simulink model "UScityblock2_Intersection"  (R2021b)
settings: Solver=ode23s  StartTime=0.0  StopTime=25  RelTol=1e-3
model workspace (MAT data in the model file):
  firstWarning = 1
  originalScenarioChecksum = '44EB4239245A86A3DA7E3FEB76A9F5A7'
values from neighbouring files (symbols this model uses):
  curvature = (DX.*D2Y - DY.*D2X) ./(DX.^2+DY.^2).^(3/2)    [setUpModel_UScityblock2.m]
  direction = ones(length(gradbp),1)    [setUpModel_UScityblock2.m]
  gradbp = linspace(0,totalDistance,50)    [setUpModel_UScityblock2.m]
  psi_o = thetaRefab(1)*(pi/180)    [setUpModel_UScityblock2.m]
  speed_actor1_gdps = smooth(speedgradbpactor1,speedactor1le)    [velocity_profiles.m]
  speed_actor2_gdps = smooth(speedgradbpactor2,speedactor2le)    [velocity_profiles.m]
  speed_actor3_gdps = smooth(speedgradbpactor3,speedactor3le)    [velocity_profiles.m]
  speed_actor4_gdps = smooth(speedgradbpactor4,speedactor4le)    [velocity_profiles.m]
  speed_ego_gdps = smooth(speedgradbpego,speedegole)    [velocity_profiles.m]
  thetaRefab = zeros(length(gradbp),1)    [setUpModel_UScityblock2.m]
  x_gdps = smooth(gradbp,xwaypoints)    [setUpModel_UScityblock2.m]
  X_o = x_ego_i(1)    [setUpModel_UScityblock2.m]
  y_gdps = smooth(gradbp,ywaypoints)    [setUpModel_UScityblock2.m]
  Y_o = y_ego_i(1)    [setUpModel_UScityblock2.m]
undefined symbols (not defined in the file or in its folder): distancecovered, gradbpA1, gradbpA2, gradbpA3, gradbpA4, gradbpego, magnitude, n, q11, v2xCA
libraries: drivingscenarioandsensors x7, sim3dautolib x5, vehdynlibtirecommon x4, autolibutils x4, aerolibconvert2 x2, simulink_extras x2, drivingvehiclecontroller x2, sim3dlib x1, vehdynlibtire x1, simulink x1, autolibshared x1
(part 1 of 2)
settings Model: Creator=REHAN  LastModifiedBy=REHAN

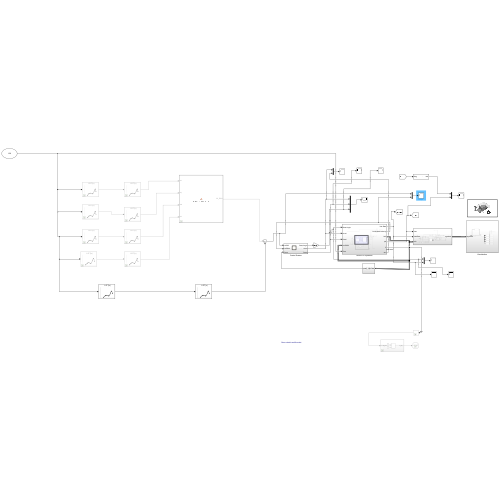
[thumbnail: Simulink's stored preview of the top-level diagram]
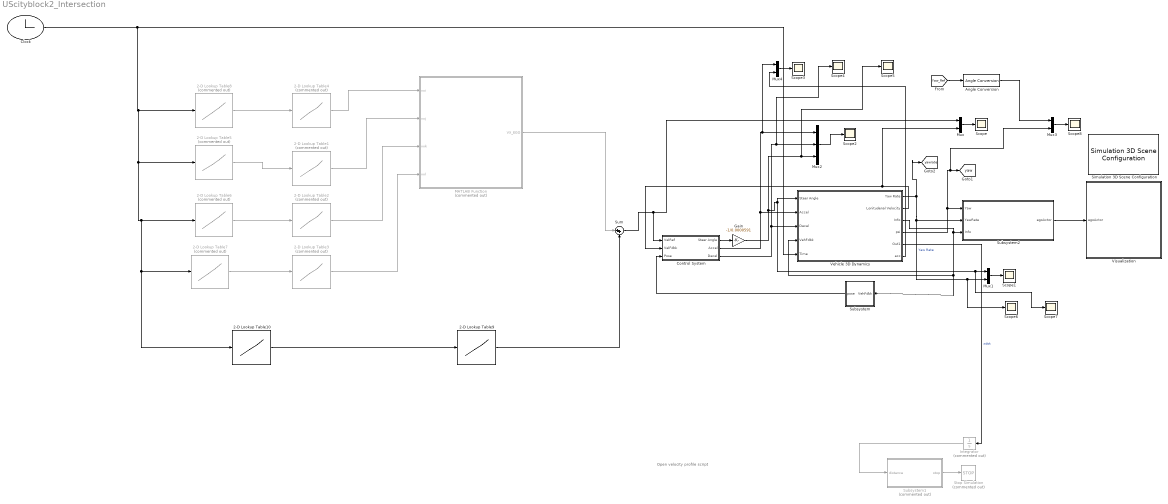
== system UScityblock2_Intersection ==
  note: Open velocity profile script
  2-D Lookup Table1 : Lookup_n-D  Commented=on  NumberOfTableDimensions=1  BreakpointsForDimension1=gradbpA1  BreakpointsForDimension2=q11(:,2)  Table=speed_actor1_gdps  InterpMethod=Cubic spline  InternalRulePriority=Speed  RndMeth=Simplest  InputSameDT=on
  2-D Lookup Table10 : Lookup_n-D  NumberOfTableDimensions=1  BreakpointsForDimension1=n  BreakpointsForDimension2=q11(:,2)  Table=gradbpego  InterpMethod=Cubic spline  InternalRulePriority=Speed  OutDataTypeStr=Inherit: Inherit from 'Table data'  RndMeth=Simplest  InputSameDT=on
  2-D Lookup Table2 : Lookup_n-D  Commented=on  NumberOfTableDimensions=1  BreakpointsForDimension1=gradbpA2  BreakpointsForDimension2=q11(:,2)  Table=speed_actor2_gdps  InterpMethod=Cubic spline  InternalRulePriority=Speed  RndMeth=Simplest  InputSameDT=on
  2-D Lookup Table3 : Lookup_n-D  Commented=on  NumberOfTableDimensions=1  BreakpointsForDimension1=gradbpA3  BreakpointsForDimension2=q11(:,2)  Table=speed_actor3_gdps  InterpMethod=Cubic spline  InternalRulePriority=Speed  RndMeth=Simplest  InputSameDT=on
  2-D Lookup Table4 : Lookup_n-D  Commented=on  NumberOfTableDimensions=1  BreakpointsForDimension1=gradbpA4  BreakpointsForDimension2=q11(:,2)  Table=speed_actor4_gdps  InterpMethod=Cubic spline  InternalRulePriority=Speed  RndMeth=Simplest  InputSameDT=on
  2-D Lookup Table5 : Lookup_n-D  Commented=on  NumberOfTableDimensions=1  BreakpointsForDimension1=n  BreakpointsForDimension2=q11(:,2)  Table=gradbpA1  InterpMethod=Cubic spline  InternalRulePriority=Speed  RndMeth=Simplest  InputSameDT=on
  2-D Lookup Table6 : Lookup_n-D  Commented=on  NumberOfTableDimensions=1  BreakpointsForDimension1=n  BreakpointsForDimension2=q11(:,2)  Table=gradbpA2  InterpMethod=Cubic spline  InternalRulePriority=Speed  RndMeth=Simplest  InputSameDT=on
  2-D Lookup Table7 : Lookup_n-D  Commented=on  NumberOfTableDimensions=1  BreakpointsForDimension1=n  BreakpointsForDimension2=q11(:,2)  Table=gradbpA3  InterpMethod=Cubic spline  InternalRulePriority=Speed  RndMeth=Simplest  InputSameDT=on
  2-D Lookup Table8 : Lookup_n-D  Commented=on  NumberOfTableDimensions=1  BreakpointsForDimension1=n  BreakpointsForDimension2=q11(:,2)  Table=gradbpA4  InterpMethod=Cubic spline  InternalRulePriority=Speed  RndMeth=Simplest  InputSameDT=on
  2-D Lookup Table9 : Lookup_n-D  NumberOfTableDimensions=1  BreakpointsForDimension1=gradbpego  BreakpointsForDimension2=q11(:,2)  Table=v2xCA  InterpMethod=Cubic spline  InternalRulePriority=Speed  OutDataTypeStr=Inherit: Inherit from 'Table data'  RndMeth=Simplest  InputSameDT=on
  Angle Conversion : aerolibconvert2/Angle Conversion  IU=deg  OU=rad
  Clock : Clock
  Control System : Subsystem
  Gain : Gain  Gain=-1/0.0000591
  Integrator : Integrator  Commented=on  InitialCondition=sqrt((X_o).^2+(Y_o).^2)
  MATLAB Function : MATLAB Function  Commented=on  TreatAsAtomicUnit=on
  Mux{,1,3..4} (4 alike) : Mux  Inputs=2
  Mux2 : Mux  Inputs=3
  Scope{,1..8} (9 alike) : Scope
  Simulation 3D Scene Configuration : sim3dlib/Simulation 3D Scene Configuration  Priority=0  ProjectFormat_internal=Default Scenes  ProjectFormat=Default Scenes  SceneDesc=US city block  ProjectName=C:\Program Files\MATLAB\R2021b\toolbox\shared\sim3d_projects\automotive_project\UE4\WindowsNoEditor\VehicleSimulation.exe  ScenePath=/Game/Maps/HwStrght  vehTagList={'Scene Origin';'SimulinkVehicle1';'SimulinkVehicle2';'SimulinkVehicle3';'SimulinkVehicle4';'SimulinkVehicle5'}  vehTag=SimulinkVehicle1  OpVisEn=off  Ts=1/60  EnableWindow=off  EnableWeather=off  SunAltitude=40.0  SunAzimuth=90  clouds=10  wind=1  fog=0  rain=79.0  sensorTag=MainCamera1  sensorId=1  sensorName=MainCamera1  mountLoc=Origin  offsetFlag=off  tmountOffset=[0, 0, 0]  rmountOffset=[0, 0, 0]  HorizontalResolution=1280  VerticalResolution=720  HorizontalFOV=60  mountPoint=[0 0 0]  mountOrientation=[0 0 0]  aMode=3  ID=1
      settings: SourceProductBaseCode=AE,DR,UV,VE
  Stop Simulation : Stop  Commented=on
  Subsystem : Subsystem
  Subsystem1 : Subsystem  Commented=on
  Subsystem2 : Subsystem
  Sum : Sum  Inputs=|++
  Vehicle 3D Dynamics : Subsystem
  "Visualization " : Subsystem
  tag scope: yaw=global, yawrate=global
  wires:
  Subsystem2/1(egoActor) -> "Visualization "/1(egoActor)
  Vehicle 3D Dynamics/3(Info) -> Subsystem/1(VehFdbk), Vehicle 3D Dynamics/4(VehFdbk), Subsystem2/3(Info)
  Vehicle 3D Dynamics/1(Yaw Rate) -> Scope6/1, Mux1/2, Subsystem2/2(YawRate), [yawrate]  "Yaw Rate"
  Vehicle 3D Dynamics/4(psi) -> Mux3/2, [yaw], Subsystem2/1(Yaw)
  Vehicle 3D Dynamics/2(Lonitudenal Velocity) -> Mux/2, Control System/2(VelFdbk)
  Subsystem/1(pose) -> Control System/3(Pose)
  Control System/1(Steer Angle) -> Gain/1
  Control System/2(Accel) -> Mux4/1, Mux2/1, Vehicle 3D Dynamics/2(Accel)
  Control System/3(Decel) -> Scope4/1, Mux2/2, Vehicle 3D Dynamics/3(Decel)
  Mux/1 -> Scope/1
  Mux1/1 -> Scope1/1
  Mux2/1 -> Scope2/1
  [Yaw_Ref] -> Angle Conversion/1
  Mux3/1 -> Scope8/1
  Integrator/1 -> Subsystem1/1(distance)
  Subsystem1/1(stop) -> Stop Simulation/1
  Vehicle 3D Dynamics/5(Out1) -> Integrator/1  "xdot"
  Angle Conversion/1 -> Mux3/1
  Vehicle 3D Dynamics/6(acc) -> Mux4/2
  Mux4/1 -> Scope3/1
  Sum/1 -> Mux/1, Control System/1(VelRef)
  2-D Lookup Table1/1 -> MATLAB Function/2(vxj)
  2-D Lookup Table2/1 -> MATLAB Function/3(vxk)
  2-D Lookup Table3/1 -> MATLAB Function/4(vxl)
  2-D Lookup Table4/1 -> MATLAB Function/1(vxi)
  2-D Lookup Table8/1 -> 2-D Lookup Table4/1
  2-D Lookup Table5/1 -> 2-D Lookup Table1/1
  2-D Lookup Table6/1 -> 2-D Lookup Table2/1
  2-D Lookup Table7/1 -> 2-D Lookup Table3/1
  Clock/1 -> Vehicle 3D Dynamics/5(Time), 2-D Lookup Table10/1, 2-D Lookup Table7/1, 2-D Lookup Table6/1, 2-D Lookup Table5/1, 2-D Lookup Table8/1
  MATLAB Function/1(VX_EGO) -> Sum/1
  2-D Lookup Table9/1 -> Sum/2
  2-D Lookup Table10/1 -> 2-D Lookup Table9/1
  Gain/1 -> Scope5/1, Mux2/3, Scope7/1, Mux1/1, Vehicle 3D Dynamics/1(Steer Angle)

== system UScityblock2_Intersection/Control System ==
  note: Controller
  VelRef : Inport
  VelFdbk : Inport  Port=2
  Pose : Inport  Port=3
  Stanley Based Controller : Subsystem  VariantControl=Stanley
  Steer Angle : Outport
  Accel : Outport  Port=2
  Decel : Outport  Port=3
  wires:
  VelFdbk/1 -> Stanley Based Controller/3(VelFdbk)
  Pose/1 -> Stanley Based Controller/1(Pose)
  Stanley Based Controller/3(DecelCmd) -> Decel/1  "Decel"
  Stanley Based Controller/2(AccelCmd) -> Accel/1  "Accel"
  Stanley Based Controller/1(WheelSteeringAngle) -> Steer Angle/1  "Steer Angle"
  VelRef/1 -> Stanley Based Controller/2(VelRef)

== system UScityblock2_Intersection/Subsystem ==
  VehFdbk : Inport
  Bus Selector : BusSelector  OutputSignals=InertFrm.Cg.Disp.X,InertFrm.Cg.Disp.Y,InertFrm.Cg.Ang.psi
  Gain1 : Gain  Gain=180/pi
  Mux : Mux  Inputs=3
  Transpose : Math  Operator=transpose  SignedPower=on  SaturateOnIntegerOverflow=on
  pose : Outport
  wires:
  Mux/1 -> Transpose/1
  VehFdbk/1 -> Bus Selector/1
  Bus Selector/1 -> Mux/1  "<X>"
  Gain1/1 -> Mux/3
  Bus Selector/2 -> Mux/2  "<Y>"
  Transpose/1 -> pose/1
  Bus Selector/3 -> Gain1/1  "<psi>"

== system UScityblock2_Intersection/Subsystem1 ==
  distance : Inport
  Constant : Constant
  Constant3 : Constant  Value=0
  Switch : Switch  Threshold=distancecovered-10
  stop : Outport
  wires:
  Switch/1 -> stop/1
  Constant3/1 -> Switch/3
  distance/1 -> Switch/2
  Constant/1 -> Switch/1

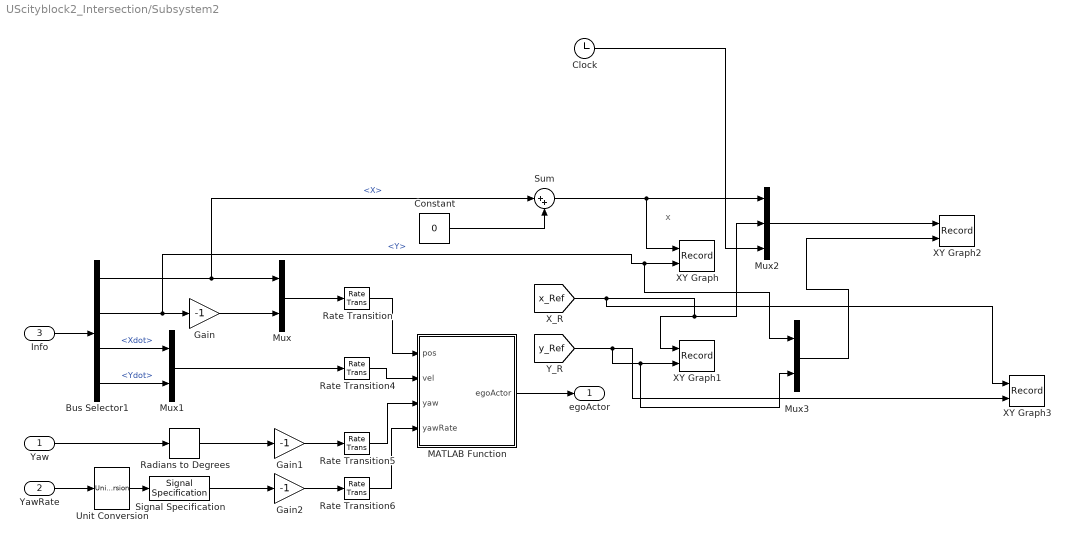
== system UScityblock2_Intersection/Subsystem2 ==
  note: x
  Yaw : Inport
  YawRate : Inport  Port=2
  Info : Inport  Port=3
  Bus Selector1 : BusSelector  OutputSignals=InertFrm.Cg.Disp.X,InertFrm.Cg.Disp.Y,InertFrm.Cg.Vel.Xdot,InertFrm.Cg.Vel.Ydot
  Clock : Clock
  Constant : Constant  Value=0
  Gain : Gain  Gain=-1
  Gain1 : Gain  Gain=-1
  Gain2 : Gain  Gain=-1
  MATLAB Function : MATLAB Function  TreatAsAtomicUnit=on
  Mux : Mux  Inputs=2
  Mux1 : Mux  Inputs=2
  Mux2 : Mux  Inputs=3
  Mux3 : Mux  Inputs=2
  Radians to Degrees : simulink_extras/Transformations/Radians to Degrees
  Rate Transition{,4..6} (4 alike) : RateTransition
  Signal Specification : SignalSpecification  Unit=deg/s
  Sum : Sum  Inputs=|++
  Unit Conversion : UnitConversion
  XY Graph : Record  FileSettingsInternal="{\"entries\":[{\"content\":{\"excelSettings\":{\"content\":{},\"type\":\"Streamout.ExcelSettings\"}},\"type\":\"Streamout.FileSettingStorage\",\"uuid\":\"01a8cffc-2acb-4a4a-b155-81213efd3857\"}],\"packageUris\":[\"http://schema.mathworks.com/mf0/streamout_blocks/R2020a\"],\"version\":\"1.0\"}"  Layout=[1 1]  SignalsInternal="{\"entries\":[{\"content\":{\"signals\":[{\"content\":{\"blockPath\":[\"UScityblock2_Intersection/Subsystem2/XY Graph\"],\"channel\":[],\"dimensions\":[1],\"domain\":\"UScityblock2_Intersection/Subsystem2/XY Graph\",\"lineColor\":\"#22b573\",\"plots\":[1],\"port\":1,\"sid\":[\"\"],\"signalID\":236514,\"signalName\":\"Sum\"},\"type\":\"RecordBlkView.Signal\",\"uuid\":\"2facecf0-700f-4d84-9e53-88a16c1cf5c3\"},{\"content\":{\"blockPath\":[\"UScityblock2_Intersection/Subsystem2/XY Graph\"],\"channel\":[],\"dimensions\":[1],\"domain\":\"UScityblock2_Intersection/Subsystem2/XY Graph\",\"lineColor\":\"#0072bd\",\"plots\":[1],\"port\":2,\"sid\":[\"\"],\"signalID\":236518,\"signalName\":\"<Y>\"},\"type\":\"RecordBlkView.Signal\",\"uuid\":\"dd458366-3161-4431-b8ca-c66b7bf56a27\"}]},\"type\":\"RecordBlkView.InputSignals\",\"uuid\":\"0316f84a-9abb-4d81-892a-fffad983f299\"}],\"packageUris\":[\"http://schema.mathworks.com/mf0/streamout_blocks/R2020a\"],\"version\":\"1.0\"}"  VisualizationBindings="{\"xyplotplugin\":{\"info\":[{\"series\":[{\"bindingParametersList\":[{\"parameter\":\"X-Axis\",\"signalID\":236514,\"signalName\":\"Sum\"},{\"parameter\":\"Y-Axis\",\"signalID\":236518,\"signalName\":\"<Y>\"}],\"seriesID\":1562}],\"subplotID\":1}]}}"  CompatibilityTag=XY
  XY Graph1 : Record  FileSettingsInternal="{\"entries\":[{\"content\":{\"excelSettings\":{\"content\":{},\"type\":\"Streamout.ExcelSettings\"}},\"type\":\"Streamout.FileSettingStorage\",\"uuid\":\"65194316-61b3-4cf9-8b54-50b4f08b8558\"}],\"packageUris\":[\"http://schema.mathworks.com/mf0/streamout_blocks/R2020a\"],\"version\":\"1.0\"}"  Layout=[1 1]  SignalsInternal="{\"entries\":[{\"content\":{\"signals\":[{\"content\":{\"blockPath\":[\"UScityblock2_Intersection/Subsystem2/XY Graph1\"],\"channel\":[],\"dimensions\":[1],\"domain\":\"UScityblock2_Intersection/Subsystem2/XY Graph1\",\"lineColor\":\"#d95319\",\"plots\":[1],\"port\":1,\"sid\":[\"\"],\"signalID\":236522,\"signalName\":\"X_R\"},\"type\":\"RecordBlkView.Signal\",\"uuid\":\"d769c5ff-0305-4b5e-81d5-133ef8863508\"},{\"content\":{\"blockPath\":[\"UScityblock2_Intersection/Subsystem2/XY Graph1\"],\"channel\":[],\"dimensions\":[1],\"domain\":\"UScityblock2_Intersection/Subsystem2/XY Graph1\",\"lineColor\":\"#edb120\",\"plots\":[1],\"port\":2,\"sid\":[\"\"],\"signalID\":236526,\"signalName\":\"Y_R\"},\"type\":\"RecordBlkView.Signal\",\"uuid\":\"f028ea11-a031-4a8e-b6b5-1ddc8b9f1194\"}]},\"type\":\"RecordBlkView.InputSignals\",\"uuid\":\"7a411283-c608-4123-8a2d-0518ba73f414\"}],\"packageUris\":[\"http://schema.mathworks.com/mf0/streamout_blocks/R2020a\"],\"version\":\"1.0\"}"  VisualizationBindings="{\"xyplotplugin\":{\"info\":[{\"series\":[{\"bindingParametersList\":[{\"parameter\":\"X-Axis\",\"signalID\":236522,\"signalName\":\"X_R\"},{\"parameter\":\"Y-Axis\",\"signalID\":236526,\"signalName\":\"Y_R\"}],\"seriesID\":23516}],\"subplotID\":1}]}}"  CompatibilityTag=XY
  XY Graph2 : Record  FileSettingsInternal="{\"entries\":[{\"content\":{\"excelSettings\":{\"content\":{},\"type\":\"Streamout.ExcelSettings\"}},\"type\":\"Streamout.FileSettingStorage\",\"uuid\":\"380f824c-9f71-4394-a0d5-a271a1d4312d\"}],\"packageUris\":[\"http://schema.mathworks.com/mf0/streamout_blocks/R2020a\"],\"version\":\"1.0\"}"  Layout=[1 1]  SignalsInternal="{\"entries\":[{\"content\":{\"signals\":[{\"content\":{\"blockPath\":[\"UScityblock2_Intersection/Subsystem2/XY Graph2\"],\"channel\":[],\"dimensions\":[3],\"domain\":\"UScityblock2_Intersection/Subsystem2/XY Graph2\",\"hasChildren\":true,\"lineColor\":\"#139fff\",\"plots\":[],\"port\":1,\"sid\":[\"\"],\"signalID\":236530,\"signalName\":\"Mux2\"},\"type\":\"RecordBlkView.Signal\",\"uuid\":\"df360da2-2f77-4849-a95a-fec057b1eca7\"},{\"content\":{\"blockPath\":[\"UScityblock2_Intersection/Subsystem2/XY Graph2\"],\"channel\":[1],\"dimensions\":[3],\"domain\":\"UScityblock2_Intersection/Subsystem2/XY Graph2\",\"lineColor\":\"#0072bd\",\"parentID\":236530,\"plots\":[1],\"port\":1,\"sid\":[\"\"],\"signalID\":236531,\"signalName\":\"Mux2\"},\"type\":\"RecordBlkView.Signal\",\"uuid\":\"277a6a10-9b58-49d5-b060-6453cc58bdd2\"},{\"content\":{\"blockPath\":[\"UScityblock2_Intersection/Subsystem2/XY Graph2\"],\"channel\":[],\"dimensions\":[2],\"domain\":\"UScityblock2_Intersection/Subsystem2/XY Graph2\",\"hasChildren\":true,\"lineColor\":\"#b746ff\",\"plots\":[],\"port\":2,\"sid\":[\"\"],\"signalID\":236535,\"signalName\":\"Mux3\"},\"type\":\"RecordBlkView.Signal\",\"uuid\":\"e9884f0a-07a4-419e-8a6f-ea5add28b795\"},{\"content\":{\"blockPath\":[\"UScityblock2_Intersection/Subsystem2/XY Graph2\"],\"channel\":[1],\"dimensions\":[2],\"domain\":\"UScityblock2_Intersection/Subsystem2/XY Graph2\",\"lineColor\":\"#edb120\",\"parentID\":236535,\"plots\":[1],\"port\":2,\"sid\":[\"\"],\"signalID\":236536,\"signalName\":\"Mux3\"},\"type\":\"RecordBlkView.Signal\",\"uuid\":\"0f214156-f115-4f05-ace6-a349634ed3a1\"},{\"content\":{\"blockPath\":[\"UScityblock2_Intersection/Subsystem2/XY Graph2\"],\"channel\":[2],\"dimensions\":[3],\"domain\":\"UScityblock2_Intersection/Subsystem2/XY Graph2\",\"lineColor\":\"#64d413\",\"parentID\":236530,\"plots\":[1],\"port\":1,\"sid\":[\"\"],\"signalID\":237249,\"signalName\":\"Mux2\"},\"type\":\"RecordBlkView.Signal\",\"uuid\":\"71064ab1-1239-4248-9448-1e7b0206ca40\"},{\"content\":{\"blockPath\":[\"UScityblock2_Intersection/Subsystem2/XY Graph2\"],\"channel\":[3],\"dimensions\":[3],\"domain\":\"UScityblock2_Intersection/Subsystem2/XY Graph2\",\"lineColor\":\"#ff13a6\",\"parentID\":236530,\"plots\":[],\"port\":1,\"sid\":[\"\"],\"signalID\":237250,\"signalName\":\"Mux2\"},\"type\":\"RecordBlkView.Signal\",\"uuid\":\"dc83131f-e559-478c-a597-548131086460\"},{\"content\":{\"blockPath\":[\"UScityblock2_Intersection/Subsystem2/XY Graph2\"],\"channel\":[2],\"dimensions\":[2],\"domain\":\"UScityblock2_Intersection/Subsystem2/XY Graph2\",\"lineColor\":\"#fe330a\",\"parentID\":236535,\"plots\":[1],\"port\":2,\"sid\":[\"\"],\"signalID\":237251,\"signalName\":\"Mux3\"},\"type\":\"RecordBlkView.Signal\",\"uuid\":\"12f8cf5f-aafd-4b0d-b784-9572c82a3249\"}]},\"type\":\"RecordBlkView.InputSignals\",\"uuid\":\"fdfec471-d303-4ed7-aee6-e58bc8732c46\"}],\"packageUris\":[\"http://schema.mathworks.com/mf0/streamout_blocks/R2020a\"],\"version\":\"1.0\"}"  VisualizationBindings="{\"xyplotplugin\":{\"info\":[{\"series\":[{\"bindingParametersList\":[{\"parameter\":\"X-Axis\",\"signalID\":236536,\"signalName\":\"Mux3(1)\"},{\"parameter\":\"Y-Axis\",\"signalID\":237251,\"signalName\":\"Mux3(2)\"}],\"seriesID\":41366},{\"bindingParametersList\":[{\"parameter\":\"X-Axis\",\"signalID\":236531,\"signalName\":\"Mux2(1)\"},{\"parameter\":\"Y-Axis\",\"signalID\":237249,\"signalName\":\"Mux2(2)\"}],\"seriesID\":18903}],\"subplotID\":1}]}}"  CompatibilityTag=XY
  XY Graph3 : Record  FileSettingsInternal="{\"entries\":[{\"content\":{\"excelSettings\":{\"content\":{},\"type\":\"Streamout.ExcelSettings\"}},\"type\":\"Streamout.FileSettingStorage\",\"uuid\":\"e705e1b1-bfa7-4bf8-b6a6-8f7c7fd2f61e\"}],\"packageUris\":[\"http://schema.mathworks.com/mf0/streamout_blocks/R2020a\"],\"version\":\"1.0\"}"  Layout=[1 1]  SignalsInternal="{\"entries\":[{\"content\":{\"signals\":[{\"content\":{\"blockPath\":[\"UScityblock2_Intersection/Subsystem2/XY Graph3\"],\"channel\":[],\"dimensions\":[1],\"domain\":\"UScityblock2_Intersection/Subsystem2/XY Graph3\",\"lineColor\":\"#a2142f\",\"plots\":[1],\"port\":1,\"sid\":[\"\"],\"signalID\":236540,\"signalName\":\"X_R\"},\"type\":\"RecordBlkView.Signal\",\"uuid\":\"8dd93952-cce1-44da-93c4-9db5071bcf04\"},{\"content\":{\"blockPath\":[\"UScityblock2_Intersection/Subsystem2/XY Graph3\"],\"channel\":[],\"dimensions\":[1],\"domain\":\"UScityblock2_Intersection/Subsystem2/XY Graph3\",\"lineColor\":\"#139fff\",\"plots\":[1],\"port\":2,\"sid\":[\"\"],\"signalID\":236544,\"signalName\":\"Y_R\"},\"type\":\"RecordBlkView.Signal\",\"uuid\":\"8d537924-d463-4c82-af9e-d2ae47232ef7\"}]},\"type\":\"RecordBlkView.InputSignals\",\"uuid\":\"02082c9e-38c5-410c-a88c-63a160a95658\"}],\"packageUris\":[\"http://schema.mathworks.com/mf0/streamout_blocks/R2020a\"],\"version\":\"1.0\"}"  VisualizationBindings="{\"xyplotplugin\":{\"info\":[{\"series\":[{\"bindingParametersList\":[{\"parameter\":\"X-Axis\",\"signalID\":236540,\"signalName\":\"X_R\"},{\"parameter\":\"Y-Axis\",\"signalID\":236544,\"signalName\":\"Y_R\"}],\"seriesID\":18086}],\"subplotID\":1}]}}"  CompatibilityTag=XY
  egoActor : Outport
  wires:
  Mux/1 -> Rate Transition/1
  Rate Transition/1 -> MATLAB Function/1(pos)
  Rate Transition4/1 -> MATLAB Function/2(vel)
  Signal Specification/1 -> Gain2/1
  Bus Selector1/4 -> Mux1/2  "<Ydot>"
  Rate Transition5/1 -> MATLAB Function/3(yaw)
  Rate Transition6/1 -> MATLAB Function/4(yawRate)
  Bus Selector1/1 -> Sum/1, Mux/1  "<X>"
  Mux1/1 -> Rate Transition4/1
  YawRate/1 -> Unit Conversion/1
  Yaw/1 -> Radians to Degrees/1
  Radians to Degrees/1 -> Gain1/1
  Info/1 -> Bus Selector1/1
  Gain2/1 -> Rate Transition6/1
  Unit Conversion/1 -> Signal Specification/1
  Gain1/1 -> Rate Transition5/1
  Bus Selector1/3 -> Mux1/1  "<Xdot>"
  MATLAB Function/1(egoActor) -> egoActor/1
  [x_Ref] -> XY Graph3/1, XY Graph1/1, Mux2/2
  Gain/1 -> Mux/2
  [y_Ref] -> XY Graph3/2, XY Graph1/2, Mux3/2
  Mux2/1 -> XY Graph2/1
  Mux3/1 -> XY Graph2/2
  Bus Selector1/2 -> Mux3/1, XY Graph/2, Gain/1  "<Y>"
  Sum/1 -> XY Graph/1, Mux2/1
  Constant/1 -> Sum/2
  Clock/1 -> Mux2/3

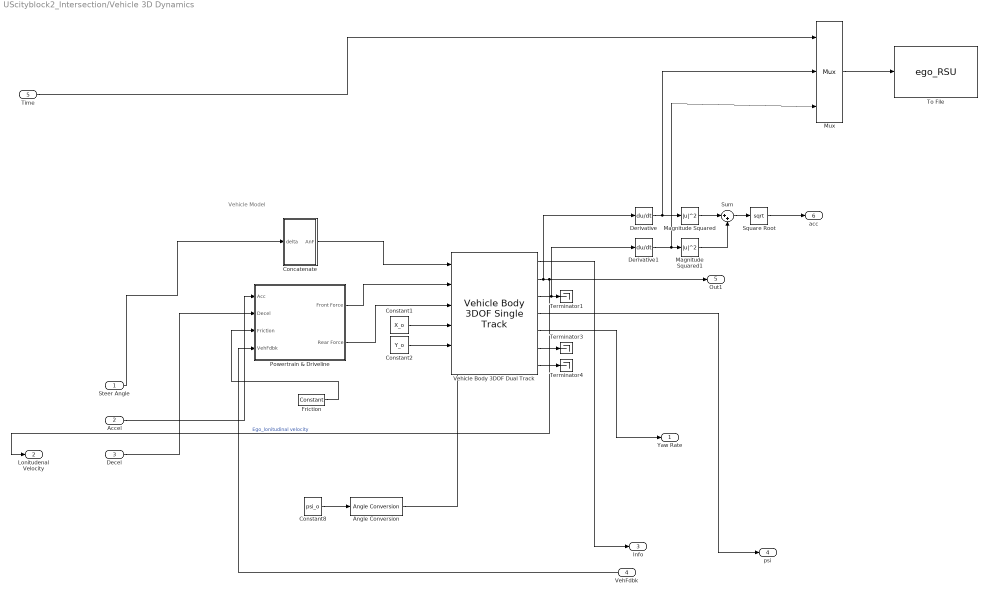
== system UScityblock2_Intersection/Vehicle 3D Dynamics ==
  note: Vehicle Model
  Steer Angle : Inport
  Accel : Inport  Port=2
  Decel : Inport  Port=3
  VehFdbk : Inport  Port=4
  Time : Inport  Port=5
  Angle Conversion : aerolibconvert2/Angle Conversion  IU=rad  OU=deg
  Concatenate : Subsystem
  Constant1 : Constant  Value=X_o
  Constant2 : Constant  Value=Y_o
  Constant8 : Constant  Value=psi_o
  Derivative : Derivative
  Derivative1 : Derivative
  Friction : vehdynlibtirecommon/Constant  const=1  numWheels=4
      settings: SourceProductBaseCode=VE
  Magnitude Squared : Math  Operator=magnitude^2  SaturateOnIntegerOverflow=on
  Magnitude Squared1 : Math  Operator=magnitude^2  SaturateOnIntegerOverflow=on
  Mux : Mux  Inputs=3
  Powertrain & Driveline : Subsystem
      mask Display: image('vdbslibpt.png');
  Square Root : Sqrt  SaturateOnIntegerOverflow=on
  Sum : Sum  Inputs=|++
  Terminator1 : Terminator
  Terminator3 : Terminator
  Terminator4 : Terminator
  To File : ToFile  Filename=ego_RSU  MatrixName=waypointstimeseries
      settings: Decimation=100
  Vehicle Body 3DOF Dual Track : autolibshared/Vehicle Body 3DOF Single Track  trackMode=Dual  inputMode=External forces  frontSteerMode=on  rearSteerMode=off  windMode=off  muMode=off  extFMode=off  extMMode=off  htchFMode=off  htchMMode=off  extXo=on  extpsio=on  extxdoto=off  extro=off  extYo=on  extTamb=off  extydoto=off  aMode=2  NF=2  NR=2  m=2000  a=1.4  b=1.4  h=0.35  dh=1  hh=0.2  X_o=0  xdot_o=speed_ego_gdps(1)  CalphaMode=off  sigmaMode=on  d=0  hl=0  w=[1.4,1.4]  Cy_f=12e3  Cy_r=11e3  sigma_f=.1  sigma_r=.1  alpha_f_brk=[-.1 .1]  Cy_f_data=[-9e3 9e3]  alpha_r_brk=[-.1 .1]  Cy_r_data=[-9e3 9e3]  Y_o=0  ydot_o=0  Izz=1000  psi_o=0  r_o=0  Af=2  Cd=.3  Cl=.1  Cpm=.1  beta_w=[0:0.01:0.3]  Cs=[0:0.03:0.9]  Cym=[0:0.01:0.3]  Pabs=101325  Tair=273  g=9.81  mu=1  xdot_tol=.01  Fznom=5000  Fxtire_sat=7e4  Fytire_sat=7e4  longOff=0  latOff=0  vertOff=0  wrapAng=off
      settings: SourceProductBaseCode=PW,DR,MT,UV,VE
  Yaw Rate : Outport
  Lonitudenal Velocity : Outport  Port=2
  Info : Outport  Port=3
  psi : Outport  Port=4
  Out1 : Outport  Port=5
  acc : Outport  Port=6
  wires:
  Decel/1 -> Powertrain & Driveline/2(Decel)
  Constant8/1 -> Angle Conversion/1
  Vehicle Body 3DOF Dual Track/7 -> Terminator4/1
  Vehicle Body 3DOF Dual Track/1 -> Info/1
  Vehicle Body 3DOF Dual Track/6 -> Terminator3/1
  Constant2/1 -> Vehicle Body 3DOF Dual Track/5
  Powertrain & Driveline/1(Front Force) -> Vehicle Body 3DOF Dual Track/2
  Friction/1 -> Powertrain & Driveline/3(Friction)
  Vehicle Body 3DOF Dual Track/2 -> Derivative/1, Out1/1, Lonitudenal Velocity/1  "Ego_lonitudinal velocity"
  Vehicle Body 3DOF Dual Track/3 -> Derivative1/1, Terminator1/1
  Constant1/1 -> Vehicle Body 3DOF Dual Track/4
  Powertrain & Driveline/2(Rear Force) -> Vehicle Body 3DOF Dual Track/3
  Accel/1 -> Powertrain & Driveline/1(Acc)
  Vehicle Body 3DOF Dual Track/5 -> Yaw Rate/1
  Vehicle Body 3DOF Dual Track/4 -> psi/1
  VehFdbk/1 -> Powertrain & Driveline/4(VehFdbk)
  Steer Angle/1 -> Concatenate/1(delta)
  Concatenate/1(AnF) -> Vehicle Body 3DOF Dual Track/1
  Angle Conversion/1 -> Vehicle Body 3DOF Dual Track/6
  Derivative/1 -> Mux/2, Magnitude Squared/1
  Derivative1/1 -> Mux/3, Magnitude Squared1/1
  Magnitude Squared/1 -> Sum/1
  Sum/1 -> Square Root/1
  Square Root/1 -> acc/1
  Time/1 -> Mux/1
  Mux/1 -> To File/1
  Magnitude Squared1/1 -> Sum/2

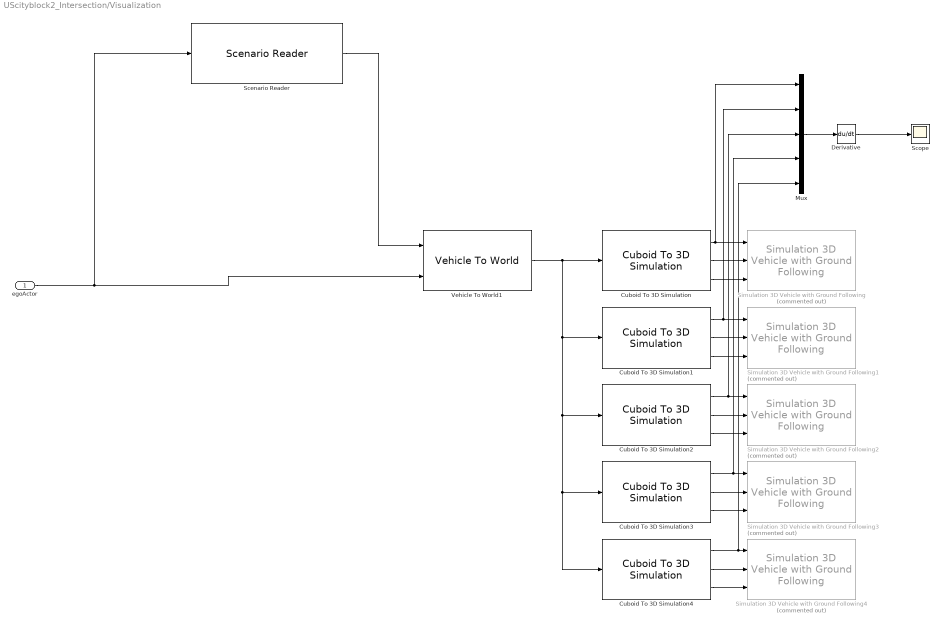
== system UScityblock2_Intersection/Visualization  ==
  egoActor : Inport
  Cuboid To 3D Simulation : drivingscenarioandsensors/Cuboid To 3D Simulation  SpecifyActorID=off  ActorIDToConvert=1  SimulateUsing=Interpreted execution
      settings: SourceProductBaseCode=DR
  Cuboid To 3D Simulation1 : drivingscenarioandsensors/Cuboid To 3D Simulation  SpecifyActorID=off  ActorIDToConvert=2  SimulateUsing=Interpreted execution
      settings: SourceProductBaseCode=DR
  Cuboid To 3D Simulation2 : drivingscenarioandsensors/Cuboid To 3D Simulation  SpecifyActorID=off  ActorIDToConvert=3  SimulateUsing=Interpreted execution
      settings: SourceProductBaseCode=DR
  Cuboid To 3D Simulation3 : drivingscenarioandsensors/Cuboid To 3D Simulation  SpecifyActorID=off  ActorIDToConvert=4  SimulateUsing=Interpreted execution
      settings: SourceProductBaseCode=DR
  Cuboid To 3D Simulation4 : drivingscenarioandsensors/Cuboid To 3D Simulation  SpecifyActorID=off  ActorIDToConvert=4  SimulateUsing=Interpreted execution
      settings: SourceProductBaseCode=DR
  Derivative : Derivative
  Mux : Mux  Inputs=5
  Scenario Reader : drivingscenarioandsensors/Scenario Reader  ScenarioSource=From file  ScenarioFileName=C:\Users\REHAN\OneDrive - The Ohio State University\UTC PNT Resilience\simulation files\USCityBlock2.mat  ScenarioVariableName=scenario  OutputCoordinateSystem=Vehicle coordinates  EgoVehicleSource=Input port  EgoVehicleActorID=1  OrientVehiclesOnRoad=on  OutputEgoVehiclePose=on  OutputEgoVehicleState=off  SampleTime=0.1  LaneBoundaryOutput=None  LaneBoundaryDistance=0:0.5:9.5  LaneBoundaryLocation=Center of lane markings  BusNameSource=Auto  BusName=BusActors  BusNumActorsSource=Scenario  BusNumActors=100  BusName2Source=Auto  BusName2=BusLaneBoundaries  BusNumLaneBoundariesSource=Scenario  BusNumLaneBoundaries=10  BusName3Source=Auto  BusName3=BusEgoActor  BusName4Source=Auto  BusName4=BusEgoState  ShowCoordinateLabels=on  SimulateUsing=Interpreted execution
  Scope : Scope
  Simulation 3D Vehicle with Ground Following : sim3dautolib/Simulation 3D Vehicle with Ground Following  Priority=-1  Commented=on  PassVehMesh=Muscle car  PassVehMesh_Internal=Muscle car  MeshPath=/MathWorksSimulation/Vehicles/Muscle/Meshes/SK_MuscleCar.SK_MuscleCar  TrackWidth=1.9  WheelBase=3  WheelRadius=0.35  VehColor=Red  VehColor_Internal=Red  InitialPos=[-150.9000,-1.8000, 0]  InitialRot=[0, 0,0.6853]  ActorName=SimulinkVehicle1  SampleTime=-1  ActorType=SimulinkVehicle  ID=1  aMode=3  ActorTag=SimulinkVehicle1  CoordinateScheme=ISO  VehLightsControl=off  HeadlightColor=[ 1, 1, 1 ]  HighBeamIntensity=100000  LowBeamIntensity=60000  HighBeamConeAngle=70  LowBeamConeAngle=70  LeftHeadlightOrientation=[ 0, 0 ]  RightHeadlightOrientation=[ 0, 0 ]  BrakelightIntensity=500  ReverselightIntensity=500  SignallightIntensity=500  SignallightPeriod=1  SignalPulseWidth=50  TransformOutportEnabled=off
      settings: SourceProductBaseCode=AE,DR,UV,VE
  Simulation 3D Vehicle with Ground Following1 : sim3dautolib/Simulation 3D Vehicle with Ground Following  Priority=-1  Commented=on  PassVehMesh=Muscle car  PassVehMesh_Internal=Muscle car  MeshPath=/MathWorksSimulation/Vehicles/Muscle/Meshes/SK_MuscleCar.SK_MuscleCar  TrackWidth=1.9  WheelBase=3  WheelRadius=0.35  VehColor=Orange  VehColor_Internal=Orange  InitialPos=[-110.9713, -28.0022, 0]  InitialRot=[0, 0, 86.1785]  ActorName=SimulinkVehicle2  SampleTime=-1  ActorType=SimulinkVehicle  ID=2  aMode=3  ActorTag=SimulinkVehicle2  CoordinateScheme=ISO  VehLightsControl=off  HeadlightColor=[ 1, 1, 1 ]  HighBeamIntensity=100000  LowBeamIntensity=60000  HighBeamConeAngle=70  LowBeamConeAngle=70  LeftHeadlightOrientation=[ 0, 0 ]  RightHeadlightOrientation=[ 0, 0 ]  BrakelightIntensity=500  ReverselightIntensity=500  SignallightIntensity=500  SignallightPeriod=1  SignalPulseWidth=50  TransformOutportEnabled=off
      settings: SourceProductBaseCode=AE,DR,UV,VE
  Simulation 3D Vehicle with Ground Following2 : sim3dautolib/Simulation 3D Vehicle with Ground Following  Priority=-1  Commented=on  PassVehMesh=Muscle car  PassVehMesh_Internal=Muscle car  MeshPath=/MathWorksSimulation/Vehicles/Muscle/Meshes/SK_MuscleCar.SK_MuscleCar  TrackWidth=1.9  WheelBase=3  WheelRadius=0.35  VehColor=Green  VehColor_Internal=Green  InitialPos=[-84.2000, 2.50, 0]  InitialRot=[0, 0, 176.7404]  ActorName=SimulinkVehicle3  SampleTime=-1  ActorType=SimulinkVehicle  ID=3  aMode=3  ActorTag=SimulinkVehicle3  CoordinateScheme=ISO  VehLightsControl=off  HeadlightColor=[ 1, 1, 1 ]  HighBeamIntensity=100000  LowBeamIntensity=60000  HighBeamConeAngle=70  LowBeamConeAngle=70  LeftHeadlightOrientation=[ 0, 0 ]  RightHeadlightOrientation=[ 0, 0 ]  BrakelightIntensity=500  ReverselightIntensity=500  SignallightIntensity=500  SignallightPeriod=1  SignalPulseWidth=50  TransformOutportEnabled=off
      settings: SourceProductBaseCode=AE,DR,UV,VE
  Simulation 3D Vehicle with Ground Following3 : sim3dautolib/Simulation 3D Vehicle with Ground Following  Priority=-1  Commented=on  PassVehMesh=Muscle car  PassVehMesh_Internal=Muscle car  MeshPath=/MathWorksSimulation/Vehicles/Muscle/Meshes/SK_MuscleCar.SK_MuscleCar  TrackWidth=1.9  WheelBase=3  WheelRadius=0.35  VehColor=Blue  VehColor_Internal=Blue  InitialPos=[-114.9284, 33.7974, 0]  InitialRot=[0, 0, 84.2930]  ActorName=SimulinkVehicle4  SampleTime=-1  ActorType=SimulinkVehicle  ID=4  aMode=3  ActorTag=SimulinkVehicle4  CoordinateScheme=ISO  VehLightsControl=off  HeadlightColor=[ 1, 1, 1 ]  HighBeamIntensity=100000  LowBeamIntensity=60000  HighBeamConeAngle=70  LowBeamConeAngle=70  LeftHeadlightOrientation=[ 0, 0 ]  RightHeadlightOrientation=[ 0, 0 ]  BrakelightIntensity=500  ReverselightIntensity=500  SignallightIntensity=500  SignallightPeriod=1  SignalPulseWidth=50  TransformOutportEnabled=off
      settings: SourceProductBaseCode=AE,DR,UV,VE
  Simulation 3D Vehicle with Ground Following4 : sim3dautolib/Simulation 3D Vehicle with Ground Following  Priority=-1  Commented=on  PassVehMesh=Muscle car  PassVehMesh_Internal=Muscle car  MeshPath=/MathWorksSimulation/Vehicles/Muscle/Meshes/SK_MuscleCar.SK_MuscleCar  TrackWidth=1.9  WheelBase=3  WheelRadius=0.35  VehColor=Red  VehColor_Internal=Red  InitialPos=[X_o, Y_o, 0]  InitialRot=[0, 0, psi_o]  ActorName=SimulinkVehicle5  SampleTime=-1  ActorType=SimulinkVehicle  ID=5  aMode=3  ActorTag=SimulinkVehicle5  CoordinateScheme=ISO  VehLightsControl=off  HeadlightColor=[ 1, 1, 1 ]  HighBeamIntensity=100000  LowBeamIntensity=60000  HighBeamConeAngle=70  LowBeamConeAngle=70  LeftHeadlightOrientation=[ 0, 0 ]  RightHeadlightOrientation=[ 0, 0 ]  BrakelightIntensity=500  ReverselightIntensity=500  SignallightIntensity=500  SignallightPeriod=1  SignalPulseWidth=50  TransformOutportEnabled=off
      settings: SourceProductBaseCode=AE,DR,UV,VE
  Vehicle To World1 : drivingscenarioandsensors/Vehicle To World  BusNameSource=Auto  BusName=BusVehicleToWorldActors  SimulateUsing=Interpreted execution
      settings: SourceProductBaseCode=DR
  wires:
  Cuboid To 3D Simulation2/3 -> Simulation 3D Vehicle with Ground Following2/3
  Cuboid To 3D Simulation/3 -> Simulation 3D Vehicle with Ground Following/3
  Vehicle To World1/1 -> Cuboid To 3D Simulation4/1, Cuboid To 3D Simulation3/1, Cuboid To 3D Simulation2/1, Cuboid To 3D Simulation1/1, Cuboid To 3D Simulation/1
  Cuboid To 3D Simulation2/1 -> Mux/3, Simulation 3D Vehicle with Ground Following2/1
  Cuboid To 3D Simulation/2 -> Simulation 3D Vehicle with Ground Following/2
  Cuboid To 3D Simulation/1 -> Mux/1, Simulation 3D Vehicle with Ground Following/1
  Cuboid To 3D Simulation2/2 -> Simulation 3D Vehicle with Ground Following2/2
  Cuboid To 3D Simulation3/2 -> Simulation 3D Vehicle with Ground Following3/2
  Cuboid To 3D Simulation3/1 -> Mux/4, Simulation 3D Vehicle with Ground Following3/1
  Cuboid To 3D Simulation3/3 -> Simulation 3D Vehicle with Ground Following3/3
  Cuboid To 3D Simulation1/3 -> Simulation 3D Vehicle with Ground Following1/3
  Cuboid To 3D Simulation1/1 -> Mux/2, Simulation 3D Vehicle with Ground Following1/1
  Cuboid To 3D Simulation1/2 -> Simulation 3D Vehicle with Ground Following1/2
  Cuboid To 3D Simulation4/1 -> Mux/5, Simulation 3D Vehicle with Ground Following4/1
  Cuboid To 3D Simulation4/2 -> Simulation 3D Vehicle with Ground Following4/2
  Cuboid To 3D Simulation4/3 -> Simulation 3D Vehicle with Ground Following4/3
  Scenario Reader/1 -> Vehicle To World1/1
  egoActor/1 -> Scenario Reader/1, Vehicle To World1/2
  Derivative/1 -> Scope/1
  Mux/1 -> Derivative/1

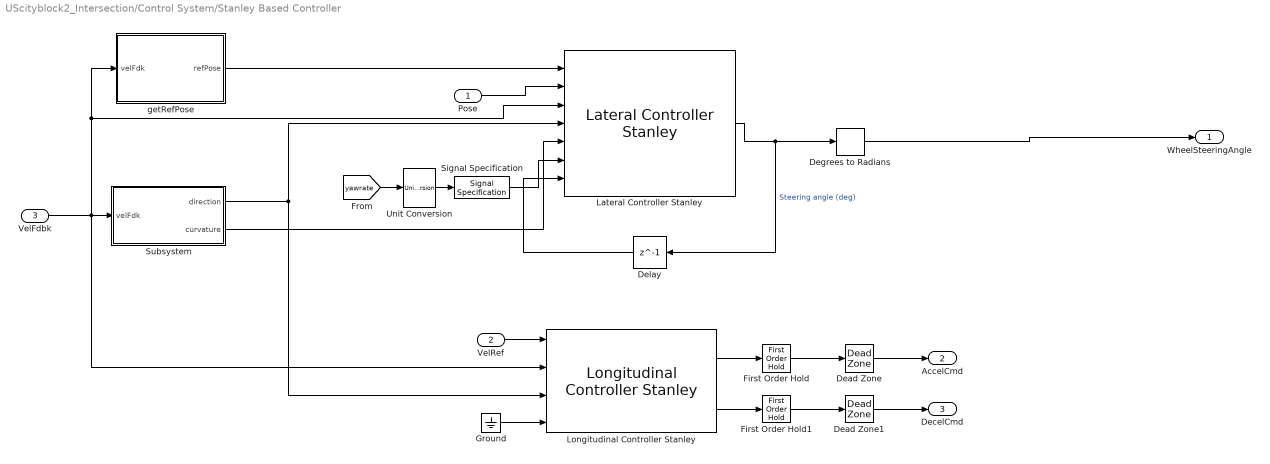
== system UScityblock2_Intersection/Control System/Stanley Based Controller ==
  Pose : Inport
  VelRef : Inport  Port=2
  VelFdbk : Inport  Port=3
  Dead Zone : DeadZone  LowerValue=-0.0001  UpperValue=0.0001  SaturateOnIntegerOverflow=on
  Dead Zone1 : DeadZone  LowerValue=-0.0001  UpperValue=0.0001  SaturateOnIntegerOverflow=on
  Degrees to Radians : simulink_extras/Transformations/Degrees to Radians
  Delay : Delay  DelayLength=1  InitialCondition=0
  First Order Hold : FirstOrderHold  ErrorTolerance=inf
  First Order Hold1 : FirstOrderHold  ErrorTolerance=inf
  Ground : Ground
  Lateral Controller Stanley : drivingvehiclecontroller/Lateral Controller Stanley  ModelType=Dynamic bicycle model  PositionGainF=0.75  PositionGainR=0.000001  YawRateGain=0.11  DelayGain=0.11  VehicleMass=2000  Lf=1.4  Lr=1.6  TireStiffness=12000  Wheelbase=3  MaxSteeringAngle=30
      settings: SourceProductBaseCode=DR
  Longitudinal Controller Stanley : drivingvehiclecontroller/Longitudinal Controller Stanley  Kp=0.75  Ki=0.12  SampleTime=0.05  MaxAcceleration=0.8  MaxDeceleration=0.8
      settings: SourceProductBaseCode=DR
  Signal Specification : SignalSpecification  Unit=deg/s
  Subsystem : Subsystem
  Unit Conversion : UnitConversion
  getRefPose : Subsystem
  WheelSteeringAngle : Outport
  AccelCmd : Outport  Port=2
  DecelCmd : Outport  Port=3
  wires:
  Longitudinal Controller Stanley/2 -> First Order Hold1/1
  VelFdbk/1 -> Longitudinal Controller Stanley/2, Subsystem/1(velFdk), getRefPose/1(velFdk), Lateral Controller Stanley/3
  Pose/1 -> Lateral Controller Stanley/2
  Ground/1 -> Longitudinal Controller Stanley/4
  Longitudinal Controller Stanley/1 -> First Order Hold/1
  getRefPose/1(refPose) -> Lateral Controller Stanley/1
  [yawrate] -> Unit Conversion/1
  Signal Specification/1 -> Lateral Controller Stanley/6
  Lateral Controller Stanley/1 -> Delay/1, Degrees to Radians/1  "Steering angle (deg)"
  Subsystem/1(direction) -> Longitudinal Controller Stanley/3, Lateral Controller Stanley/4
  VelRef/1 -> Longitudinal Controller Stanley/1
  Subsystem/2(curvature) -> Lateral Controller Stanley/5
  First Order Hold/1 -> Dead Zone/1
  First Order Hold1/1 -> Dead Zone1/1
  Dead Zone/1 -> AccelCmd/1
  Dead Zone1/1 -> DecelCmd/1
  Unit Conversion/1 -> Signal Specification/1
  Delay/1 -> Lateral Controller Stanley/7
  Degrees to Radians/1 -> WheelSteeringAngle/1

== system UScityblock2_Intersection/Vehicle 3D Dynamics/Concatenate ==
  delta : Inport
  Matrix Concatenate : Concatenate
  AnF : Outport  VectorParamsAs1DForOutWhenUnconnected=off
  tag scope: AnL=global, AnR=global
  wires:
  Matrix Concatenate/1 -> AnF/1
  delta/1 -> [AnR], Matrix Concatenate/2, Matrix Concatenate/1, [AnL]

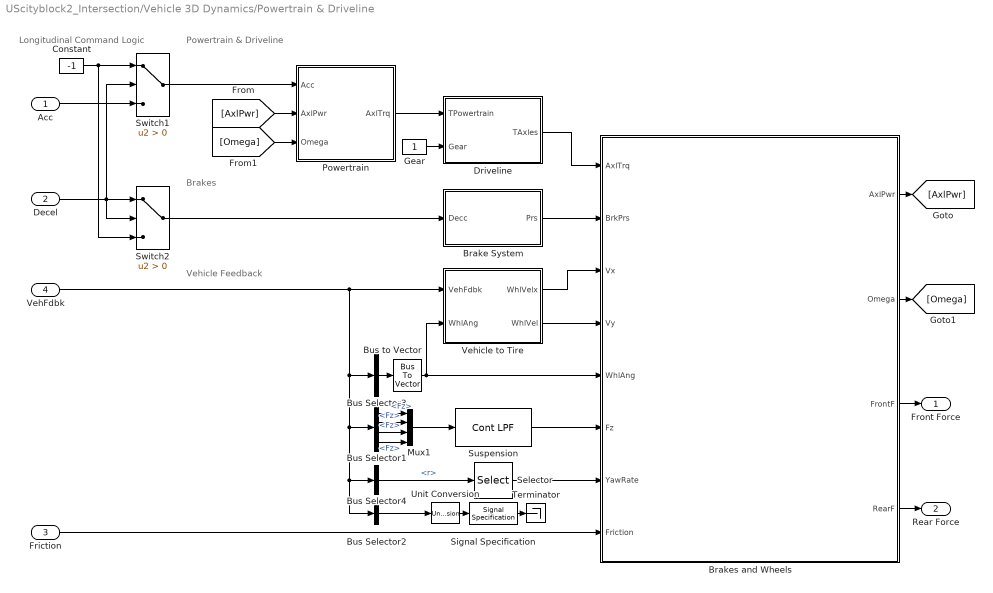
== system UScityblock2_Intersection/Vehicle 3D Dynamics/Powertrain & Driveline ==
  note: Vehicle Feedback
  note: Powertrain & Driveline
  note: Brakes
  note: Longitudinal Command Logic
  Acc : Inport
  Decel : Inport  Port=2
  Friction : Inport  Port=3
  VehFdbk : Inport  Port=4
  Brake System : Subsystem
  Brakes and Wheels : Subsystem  TreatAsAtomicUnit=on
      mask Display: image('vdbslibwhls.png');
  Bus Selector1 : BusSelector  OutputSignals=BdyFrm.Forces.Tires.FrntTires.Lft.Fz,BdyFrm.Forces.Tires.FrntTires.Rght.Fz,BdyFrm.Forces.Tires.RearTires.Lft.Fz,BdyFrm.Forces.Tires.RearTires.Rght.Fz
  Bus Selector2 : BusSelector  OutputSignals=BdyFrm.Cg.Vel.xdot  OutputAsBus=on
  Bus Selector3 : BusSelector  OutputSignals=BdyFrm.FrntAxl.Steer.WhlAngFL,BdyFrm.FrntAxl.Steer.WhlAngFR,BdyFrm.RearAxl.Steer.WhlAngRL,BdyFrm.RearAxl.Steer.WhlAngRR  OutputAsBus=on
  Bus Selector4 : BusSelector  OutputSignals=BdyFrm.Cg.AngVel.r
  Bus to Vector : BusToVector
  Constant : Constant  Value=-1
  Driveline : Subsystem  Variant=on  VariantControlMode=label  VariantControl=Variant1  LabelModeActiveChoice=0
  Gear : Constant
  Mux1 : Mux
  Powertrain : Subsystem
  Selector : Selector  InputPortWidth=1  IndexOptions=Index vector (dialog)  Indices=[1 1 1 1]  OutputSizes=1
  Signal Specification : SignalSpecification  Unit=km/hr
  Suspension : autolibutils/Cont LPF  wc=10*pi*2  aMode=2
      settings: SourceProductBaseCode=PW,DR,MT,UV,VE
  Switch1 : Switch  Criteria=u2 > Threshold
  Switch2 : Switch  Criteria=u2 > Threshold
  Terminator : Terminator
  Unit Conversion : UnitConversion
  Vehicle to Tire : Subsystem
  Front Force : Outport  VectorParamsAs1DForOutWhenUnconnected=off
  Rear Force : Outport  Port=2  VectorParamsAs1DForOutWhenUnconnected=off
  wires:
  Vehicle to Tire/2(WhlVel) -> Brakes and Wheels/4(Vy)
  Vehicle to Tire/1(WhlVelx) -> Brakes and Wheels/3(Vx)
  Brakes and Wheels/1(AxlPwr) -> [AxlPwr]
  Brakes and Wheels/4(RearF) -> Rear Force/1
  Brakes and Wheels/3(FrontF) -> Front Force/1
  Brakes and Wheels/2(Omega) -> [Omega]
  VehFdbk/1 -> Vehicle to Tire/1(VehFdbk), Bus Selector3/1, Bus Selector1/1, Bus Selector4/1, Bus Selector2/1
  Selector/1 -> Brakes and Wheels/7(YawRate)
  Bus Selector4/1 -> Selector/1  "<r>"
  Friction/1 -> Brakes and Wheels/8(Friction)
  Gear/1 -> Driveline/2(Gear)
  Signal Specification/1 -> Terminator/1
  Unit Conversion/1 -> Signal Specification/1
  Bus Selector2/1 -> Unit Conversion/1
  Brake System/1(Prs) -> Brakes and Wheels/2(BrkPrs)
  Switch2/1 -> Brake System/1(Decc)
  [Omega] -> Powertrain/3(Omega)
  [AxlPwr] -> Powertrain/2(AxlPwr)
  Powertrain/1(AxlTrq) -> Driveline/1(TPowertrain)
  Switch1/1 -> Powertrain/1(Acc)
  Bus Selector1/4 -> Mux1/4  "<Fz>"
  Bus Selector1/3 -> Mux1/3  "<Fz>"
  Bus Selector1/2 -> Mux1/2  "<Fz>"
  Bus Selector1/1 -> Mux1/1  "<Fz>"
  Suspension/1 -> Brakes and Wheels/6(Fz)
  Mux1/1 -> Suspension/1
  Bus to Vector/1 -> Brakes and Wheels/5(WhlAng), Vehicle to Tire/2(WhlAng)
  Bus Selector3/1 -> Bus to Vector/1
  Driveline/1(TAxles) -> Brakes and Wheels/1(AxlTrq)
  Constant/1 -> Switch1/1, Switch2/3
  Acc/1 -> Switch1/3
  Decel/1 -> Switch2/1, Switch2/2, Switch1/2

== system UScityblock2_Intersection/Control System/Stanley Based Controller/Subsystem ==
  velFdk : Inport
  Curvature : Lookup_n-D  NumberOfTableDimensions=1  BreakpointsForDimension1=gradbp  Table=curvature  InternalRulePriority=Speed  RndMeth=Simplest  InputSameDT=on
  Direction : Lookup_n-D  NumberOfTableDimensions=1  BreakpointsForDimension1=gradbp  Table=direction  InternalRulePriority=Speed  RndMeth=Simplest  InputSameDT=on
  Integrator1 : Integrator
  direction : Outport
  curvature : Outport  Port=2
  wires:
  velFdk/1 -> Integrator1/1
  Integrator1/1 -> Direction/1, Curvature/1
  Curvature/1 -> curvature/1
  Direction/1 -> direction/1

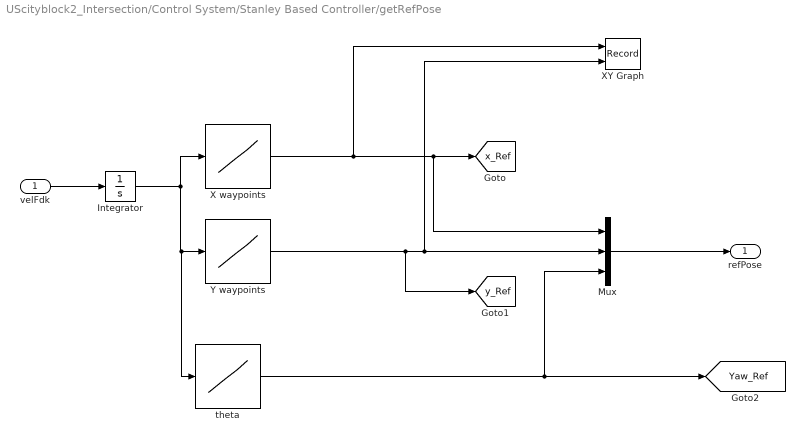
== system UScityblock2_Intersection/Control System/Stanley Based Controller/getRefPose ==
  velFdk : Inport
  Integrator : Integrator
  Mux : Mux  Inputs=3
  X waypoints : Lookup_n-D  NumberOfTableDimensions=1  BreakpointsForDimension1=gradbp  Table=x_gdps  InternalRulePriority=Speed  RndMeth=Simplest  InputSameDT=on
  XY Graph : Record  FileSettingsInternal="{\"entries\":[{\"content\":{\"excelSettings\":{\"content\":{},\"type\":\"Streamout.ExcelSettings\"}},\"type\":\"Streamout.FileSettingStorage\",\"uuid\":\"bef6bb8e-1016-4c63-aae2-f84d801cd144\"}],\"packageUris\":[\"http://schema.mathworks.com/mf0/streamout_blocks/R2020a\"],\"version\":\"1.0\"}"  Layout=[1 1]  SignalsInternal="{\"entries\":[{\"content\":{\"signals\":[{\"content\":{\"blockPath\":[\"UScityblock2_Intersection/Control System/Stanley Based Controller/getRefPose/XY Graph\"],\"channel\":[],\"dimensions\":[1],\"domain\":\"UScityblock2_Intersection/Control System/Stanley Based Controller/getRefPose/XY Graph\",\"lineColor\":\"#ff13a6\",\"plots\":[],\"port\":1,\"sid\":[\"\"],\"signalID\":236506,\"signalName\":\"X waypoints\"},\"type\":\"RecordBlkView.Signal\",\"uuid\":\"75a94f3b-5f4e-445e-b56f-92184e3f3a4b\"},{\"content\":{\"blockPath\":[\"UScityblock2_Intersection/Control System/Stanley Based Controller/getRefPose/XY Graph\"],\"channel\":[],\"dimensions\":[1],\"domain\":\"UScityblock2_Intersection/Control System/Stanley Based Controller/getRefPose/XY Graph\",\"lineColor\":\"#fe330a\",\"plots\":[],\"port\":2,\"sid\":[\"\"],\"signalID\":236510,\"signalName\":\"Y waypoints\"},\"type\":\"RecordBlkView.Signal\",\"uuid\":\"39627772-6a6c-4b55-8892-1ad78befb8e8\"}]},\"type\":\"RecordBlkView.InputSignals\",\"uuid\":\"10b3f726-df52-4ff2-a7cb-80dc495a170a\"}],\"packageUris\":[\"http://schema.mathworks.com/mf0/streamout_blocks/R2020a\"],\"version\":\"1.0\"}"  VisualizationBindings="{\"xyplotplugin\":{\"info\":[{\"series\":[],\"subplotID\":1}]}}"  CompatibilityTag=XY
  Y waypoints : Lookup_n-D  NumberOfTableDimensions=1  BreakpointsForDimension1=gradbp  Table=y_gdps  InternalRulePriority=Speed  RndMeth=Simplest  InputSameDT=on
  theta : Lookup_n-D  NumberOfTableDimensions=1  BreakpointsForDimension1=gradbp  Table=thetaRefab  InternalRulePriority=Speed  RndMeth=Simplest  InputSameDT=on
  refPose : Outport
  tag scope: Yaw_Ref=global, x_Ref=global, y_Ref=global
  wires:
  Integrator/1 -> X waypoints/1, theta/1, Y waypoints/1
  velFdk/1 -> Integrator/1
  Mux/1 -> refPose/1
  X waypoints/1 -> XY Graph/1, [x_Ref], Mux/1
  Y waypoints/1 -> [y_Ref], XY Graph/2, Mux/2
  theta/1 -> Mux/3, [Yaw_Ref]

== system UScityblock2_Intersection/Vehicle 3D Dynamics/Powertrain & Driveline/Brake System ==
  Decc : Inport
  Hydraulics : autolibutils/Cont LPF  wc=30*pi*2  aMode=2
      settings: SourceProductBaseCode=PW,DR,MT,UV,VE
  Pressure : Gain  Gain=1.5e7
  Saturation1 : Saturate  UpperLimit=inf  LowerLimit=0  ZeroCross=off
  Selector : Selector  InputPortWidth=1  IndexOptions=Index vector (dialog)  Indices=[1 1 1 1]  OutputSizes=1
  Signal Specification : SignalSpecification  Unit=Pa
  Prs : Outport  PortDimensions=4  VectorParamsAs1DForOutWhenUnconnected=off
  wires:
  Signal Specification/1 -> Prs/1
  Decc/1 -> Saturation1/1
  Selector/1 -> Signal Specification/1
  Saturation1/1 -> Hydraulics/1
  Hydraulics/1 -> Pressure/1
  Pressure/1 -> Selector/1
